simulink model "test1_AL_post"  (Simulink 8.4)
settings: Solver=ode45  StartTime=0.0  StopTime=10.0  RelTol=1e-3
settings Model: Creator=GM  LastModifiedBy=GM
settings DataIOCC: SignalLoggingSaveFormat=Dataset
settings OptimizationCC: ExpressionDepthLimit=128
settings DebuggingCC: UnderspecifiedInitializationDetection=Simplified  MergeDetectMultiDrivingBlocksExec=error  SolverPrmCheckMsg=none  FcnCallInpInsideContextMsg=EnableAllAsWarning  FrameProcessingCompatibilityMsg=error  StateNameClashWarn=none

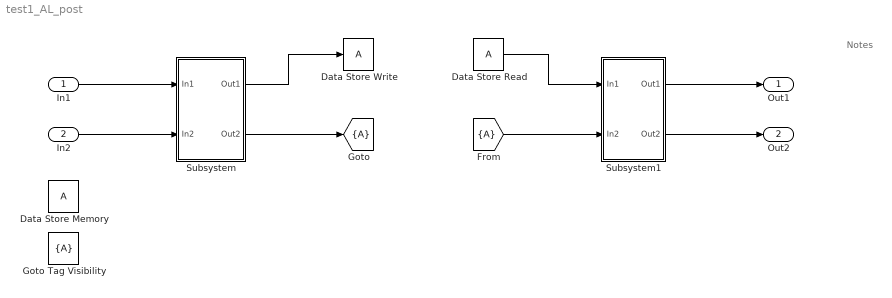
== system test1_AL_post ==
  note: Notes
  In1 : Inport
  In2 : Inport  Port=2
  Data Store Read : DataStoreRead
  Data Store Write : DataStoreWrite
  Data Store Memory : DataStoreMemory  ReadBeforeWriteMsg=warning  WriteAfterWriteMsg=warning  WriteAfterReadMsg=warning
  Goto Tag Visibility : GotoTagVisibility
  Subsystem : Subsystem
  Subsystem1 : Subsystem
  Out1 : Outport
  Out2 : Outport  Port=2
  tag scope: A=scoped
  wires:
  Subsystem/1(Out1) -> Data Store Write/1
  Subsystem/2(Out2) -> [A]
  In1/1 -> Subsystem/1(In1)
  In2/1 -> Subsystem/2(In2)
  Data Store Read/1 -> Subsystem1/1(In1)
  [A] -> Subsystem1/2(In2)
  Subsystem1/1(Out1) -> Out1/1
  Subsystem1/2(Out2) -> Out2/1

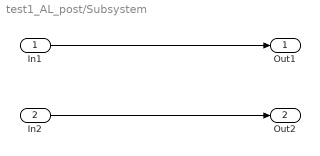
== system test1_AL_post/Subsystem ==
  In1 : Inport
  In2 : Inport  Port=2
  Out1 : Outport
  Out2 : Outport  Port=2
  wires:
  In1/1 -> Out1/1
  In2/1 -> Out2/1

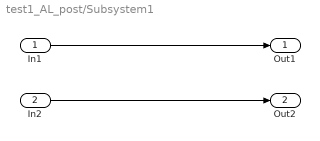
== system test1_AL_post/Subsystem1 ==
  In1 : Inport
  In2 : Inport  Port=2
  Out1 : Outport
  Out2 : Outport  Port=2
  wires:
  In1/1 -> Out1/1
  In2/1 -> Out2/1
